simulink model "DCP_DCN_PWM"  (R2013a)
settings: Solver=FixedStepDiscrete  SolverMode=SingleTasking  StartTime=0.0  StopTime=inf  FixedStep=Tpas  RelTol=1e-3
undefined symbols (not defined in the file): fmod4Q, IDCP, KLPDCP, L, Lcoup, PDCP, R, TLPDCP, Tpas, Vdc
libraries: powerlib x51, simulink x15, powerlib_meascontrol x4
settings Model: Creator=LiberT  LastModifiedBy=Francis
settings DataIOCC: SignalLoggingSaveFormat=ModelDataLogs
settings OptimizationCC: ExpressionDepthLimit=2147483647
settings DebuggingCC: MultiTaskDSMMsg=warning  MultiTaskCondExecSysMsg=none  FcnCallInpInsideContextMsg=EnableAllAsWarning  StrictBusMsg=None
settings RTWCC: IncludeERTFirstTime=on

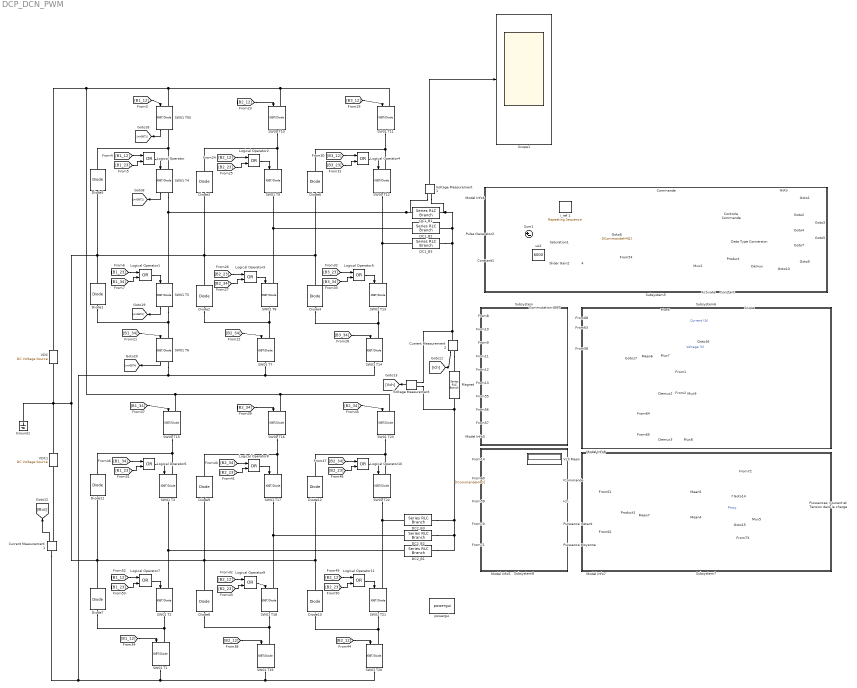
== system DCP_DCN_PWM ==
  " " : ManualSwitch
  " 4" : ManualSwitch  CurrentSetting=0
  Activate : Constant  Value=0
  Commande : Subsystem
  Commutation IGBT : Scope  NumInputPorts=9
      settings: TickLabels=on  TimeRange=0.04  YMin=-0.2~-0.2~-0.2~-0.2~-0.2~-0.2~-0.2~-0.2~-0.2  YMax=1.2~1.2~1.2~1.2~1.2~1.2~1.2~1.2~1.2
  Constant : Constant  Value=[1 1 1 1 1 1 1 1 1]
  Constant1 : Constant  Value=6000
  Controle Commande : ManualSwitch
  Current Measurement1 : powerlib/Measurements/Current Measurement  PhasorSimulation=off  OutputType=Complex  PSBequivalent=0
  Current Measurement2 : powerlib/Measurements/Current Measurement  PhasorSimulation=off  OutputType=Complex  PSBequivalent=0
  DC1_B1 : powerlib/Elements/Series RLC Branch  LConnTagsString=__new0  RConnTagsString=__new0  BranchType=L  Resistance=0  Inductance=Lcoup  SetiL0=off  InitialCurrent=0  Capacitance=1e-6  Setx0=off  InitialVoltage=0  Measurements=Branch current
  DC1_B2 : powerlib/Elements/Series RLC Branch  LConnTagsString=__new0  RConnTagsString=__new0  BranchType=L  Resistance=0  Inductance=Lcoup  SetiL0=off  InitialCurrent=0  Capacitance=1e-6  Setx0=off  InitialVoltage=0  Measurements=Branch current
  DC1_B3 : powerlib/Elements/Series RLC Branch  LConnTagsString=__new0  RConnTagsString=__new0  BranchType=L  Resistance=0  Inductance=Lcoup  SetiL0=off  InitialCurrent=0  Capacitance=1e-6  Setx0=off  InitialVoltage=0  Measurements=Branch current
  "DC2_B1 " : powerlib/Elements/Series RLC Branch  LConnTagsString=__new0  RConnTagsString=__new0  BranchType=L  Resistance=0  Inductance=Lcoup  SetiL0=off  InitialCurrent=0  Capacitance=1e-6  Setx0=off  InitialVoltage=0  Measurements=Branch current
  DC2_B2 : powerlib/Elements/Series RLC Branch  LConnTagsString=__new0  RConnTagsString=__new0  BranchType=L  Resistance=0  Inductance=Lcoup  SetiL0=off  InitialCurrent=0  Capacitance=1e-6  Setx0=off  InitialVoltage=0  Measurements=Branch current
  DC2_B3 : powerlib/Elements/Series RLC Branch  LConnTagsString=__new0  RConnTagsString=__new0  BranchType=L  Resistance=0  Inductance=Lcoup  SetiL0=off  InitialCurrent=0  Capacitance=1e-6  Setx0=off  InitialVoltage=0  Measurements=Branch current
  Data Type Conversion : DataTypeConversion  OutDataTypeStr=boolean
  Demux : Demux  Outputs=9
  Demux2 : Demux  Outputs=2
  Demux3 : Demux  Outputs=2
  Diode{1..12} (12 alike) : powerlib/Power Electronics/Diode  Ron=0.001  Lon=0  Vf=0.8  IC=0  UseSnubber=off  Rs=500  Cs=inf  Measurements=off
  Ground1 : powerlib/Elements/Ground  LConnTagsString=a
  ICommande : Display
  Ich : Display
  Logical Operator{,1..11} (12 alike) : Logic  Operator=OR  AllPortsSameDT=off  OutDataTypeStr=boolean
  Magnet : powerlib/Elements/Series RLC Branch  LConnTagsString=__new0  RConnTagsString=__new0  BranchType=RL  Resistance=R  Inductance=L  SetiL0=off  InitialCurrent=0  Capacitance=1e-6  Setx0=off  InitialVoltage=0  Measurements=Branch voltage and current
  Mean4 : powerlib_meascontrol/Measurements/Mean  Freq=1/.9  Vinit=0  Ts=Tpas
  Mean5 : powerlib_meascontrol/Measurements/Mean  Freq=fmod4Q  Vinit=0  Ts=Tpas
  Mean6 : powerlib_meascontrol/Measurements/Mean  Freq=fmod4Q/3  Vinit=0  Ts=Tpas
  Mean7 : powerlib_meascontrol/Measurements/Mean  Freq=fmod4Q/2  Vinit=0  Ts=Tpas
  Model Info{3,5,7..8} (4 alike) : simulink/Model-Wide Utilities/Model Info  InitialBlockCM=None  BlockCM=None  Frame=on  DisplayStringWithTags=Résultats  HorizontalTextAlignment=Center  LeftAlignmentValue=0.5  SourceBlockDiagram=DCP_DCN_PWM  TagMaxNumber=20
  Model Info6 : simulink/Model-Wide Utilities/Model Info  InitialBlockCM=None  BlockCM=None  Frame=on  DisplayStringWithTags=Commande H4Q  HorizontalTextAlignment=Center  LeftAlignmentValue=0.5  SourceBlockDiagram=DCP_DCN_PWM  TagMaxNumber=20
  Mux2 : Mux  Inputs=9
  Mux{5..9} (5 alike) : Mux  Inputs=2
  Product : Product
  Product1 : Product
  Puissance Instant. : Display
  Puissance Moyenne : Display
  "Puissances, Courant et Tension dans la charge" : Scope  NumInputPorts=3
      settings: TickLabels=on  TimeRange=0.9  YMin=-100~-25000000~-5000  YMax=6200~25000000~4500  SaveName=ScopeData4
  Pulse Generator2 : DiscretePulseGenerator  Amplitude=12000  Period=floor(.4 /Tpas)  PulseWidth=floor(.4 * .5 / Tpas)  PhaseDelay=floor(.001 / Tpas)  SampleTime=Tpas
  SW01 T05 : powerlib/Power Electronics/IGBT//Diode  Ron=Ron  Rs=Rs  Cs=Cs  Measurements=on
  SW01 T{1..3,7..23} (20 alike) : powerlib/Power Electronics/IGBT//Diode  Ron=Ron  Rs=Rs  Cs=Cs  Measurements=off
  SW01 T4 : powerlib/Power Electronics/IGBT//Diode  Ron=Ron  Rs=Rs  Cs=Cs  Measurements=on
  SW01 T5 : powerlib/Power Electronics/IGBT//Diode  Ron=Ron  Rs=Rs  Cs=Cs  Measurements=on
  SW01 T6 : powerlib/Power Electronics/IGBT//Diode  Ron=Ron  Rs=Rs  Cs=Cs  Measurements=on
  Saturation1 : Saturate  UpperLimit=5000  LowerLimit=2000
  Scope : Scope  NumInputPorts=6
      settings: TimeRange=0.9  YMin=-7000~-5000~-0.1~-0.1~-15000~0  YMax=7000~5000~1.1~1.1~15000~2500  SaveName=ScopeData5  MaxDataPoints=10000
  Scope1 : Scope
      settings: TimeRange=0.9  YMin=-7000  YMax=7000  SaveName=ScopeData6  MaxDataPoints=10000
  Slider Gain2 : simulink/Math Operations/Slider Gain  low=0  gain=0.54  high=1
  Subsystem : Subsystem
      mask Display: disp('')
  Subsystem5 : Subsystem
      mask Display: disp('')
  Subsystem6 : Subsystem
      mask Display: disp('')
  Subsystem7 : Subsystem
      mask Display: disp('')
  Subsystem8 : Subsystem
      mask Display: disp('')
  Sum1 : Sum  Inputs=|+-
  VDC : powerlib/Electrical Sources/DC Voltage Source  Amplitude=Vdc/2  Measurements=None
  VDC1 : powerlib/Electrical Sources/DC Voltage Source  Amplitude=Vdc/2  Measurements=None
  Vch Mean : Display
  Voltage Measurement : powerlib/Measurements/Voltage Measurement  PhasorSimulation=off  OutputType=Complex  PSBequivalent=0
  Voltage Measurement1 : powerlib/Measurements/Voltage Measurement  PhasorSimulation=off  OutputType=Complex  PSBequivalent=0
  i_ref 1 : simulink/Sources/Repeating Sequence  rep_seq_t="[0 108.51e-3 127.6e-3 132e-3 200e-3 250e-3 283.33e-3 310e-3 366.66e-3  490e-3 533e-3 683.33e-3 900e-3]"  rep_seq_y=[333 333 1000 1031 1500 2000 2500 3000 4000 6000 6000 333 333]
  powergui : powerlib/powergui  Priority=1  SimulationMode=Discrete  SolverType=Tustin  SampleTime=Tpas  frequency=60  SPID=off  DisableSnubberDevices=off  DisableRonSwitches=off  DisableVfSwitches=off  SwTol=0  Interpol=off  DisplayEquations=off  frequencyindice=0  Pbase=100e6  ErrMax=1e-4  Iterations=50  UnitsV=kV  UnitsW=MW  FunctionMessages=off  echomessages=off  HookPort=off  EnableUseOfTLC=off  x0status=blocks  RestoreLinks=warning  ResistiveCurrentMeasurement=off  Frange=[0:2:500]  Ylog=off  Xlog=on  ShowGrid=off  save=off  variable=ZData  structure=ScopeData6  ZoomFFT=off  StartTime=3.7  cycles=130  DisplayStyle=1  fundamental=333  FreqAxis=on  MaxFrequency=2000  frequencyindicesteady=1  RmsSteady=1  display=off  Ts=0  methode=off
  uo2 : Constant  Value=6000
  wires:
  [B1_12] -> Commutation IGBT/1
  [B1_23] -> Commutation IGBT/2
  [B1_34] -> Commutation IGBT/3
  [B2_12] -> Commutation IGBT/4
  [B2_23] -> Commutation IGBT/5
  [B2_34] -> Commutation IGBT/6
  Constant/1 -> Product/2
  Activate/1 -> Product/1
  Controle Commande/1 -> Demux/1
  Mux2/1 -> Controle Commande/1
  Data Type Conversion/1 -> Controle Commande/2
  Product/1 -> Data Type Conversion/1
  Commande/1(12_B1) -> Mux2/1
  Commande/2(23_B1) -> Mux2/2
  Commande/3(34_B1) -> Mux2/3
  Demux/1 -> [B1_12]
  Demux/3 -> [B1_34]
  Demux/2 -> [B1_23]
  [B1_12] -> SW01 T05/1
  Logical Operator/1 -> SW01 T4/1
  [B1_12] -> Logical Operator/1
  [B1_23] -> Logical Operator/2
  Logical Operator1/1 -> SW01 T5/1
  [B1_23] -> Logical Operator1/1
  [B1_34] -> Logical Operator1/2
  [B1_34] -> SW01 T6/1
  [B2_12] -> SW01 T10/1
  Logical Operator2/1 -> SW01 T9/1
  [B2_12] -> Logical Operator2/1
  [B2_23] -> Logical Operator2/2
  Logical Operator3/1 -> SW01 T8/1
  [B2_23] -> Logical Operator3/1
  [B2_34] -> Logical Operator3/2
  [B2_34] -> SW01 T7/1
  [B3_12] -> SW01 T11/1
  Logical Operator4/1 -> SW01 T12/1
  [B3_12] -> Logical Operator4/1
  [B3_23] -> Logical Operator4/2
  Logical Operator5/1 -> SW01 T13/1
  [B3_23] -> Logical Operator5/1
  [B3_34] -> Logical Operator5/2
  [B3_34] -> SW01 T14/1
  [B1_34] -> SW01 T15/1
  Logical Operator6/1 -> SW01 T3/1
  [B1_34] -> Logical Operator6/1
  [B1_23] -> Logical Operator6/2
  Logical Operator7/1 -> SW01 T2/1
  [B1_12] -> Logical Operator7/1
  [B1_23] -> Logical Operator7/2
  [B1_12] -> SW01 T1/1
  [B2_34] -> SW01 T16/1
  Logical Operator8/1 -> SW01 T17/1
  [B2_34] -> Logical Operator8/1
  [B2_23] -> Logical Operator8/2
  Logical Operator9/1 -> SW01 T18/1
  [B2_12] -> Logical Operator9/1
  [B2_23] -> Logical Operator9/2
  [B2_12] -> SW01 T19/1
  [B2_34] -> SW01 T23/1
  Logical Operator10/1 -> SW01 T22/1
  [B2_34] -> Logical Operator10/1
  [B2_23] -> Logical Operator10/2
  Logical Operator11/1 -> SW01 T21/1
  [B2_12] -> Logical Operator11/1
  [B2_23] -> Logical Operator11/2
  [B2_12] -> SW01 T20/1
  Current Measurement1/1 -> [IBus]
  uo2/1 -> Slider Gain2/1
  Slider Gain2/1 -> " 4"/2
  Saturation1/1 -> " 4"/1
  Constant1/1 -> Sum1/2
  i_ref 1/1 -> " "/1
  " 4"/1 -> " "/2
  Pulse Generator2/1 -> Sum1/1
  Sum1/1 -> Saturation1/1
  " "/1 -> Commande/1(Iref), [ICommandeH4Q]
  Commande/4(12_B2) -> Mux2/4
  Commande/5(23_B2) -> Mux2/5
  Commande/6(34_B2) -> Mux2/6
  Commande/7(12_B3) -> Mux2/7
  Commande/8(23_B3) -> Mux2/8
  Commande/9(34_B3) -> Mux2/9
  Demux/4 -> [B2_12]
  Demux/6 -> [B2_34]
  Demux/5 -> [B2_23]
  Demux/7 -> [B3_12]
  Demux/9 -> [B3_34]
  Demux/8 -> [B3_23]
  Current Measurement2/1 -> [Ich]
  Voltage Measurement/1 -> [Vch]
  [Ich] -> Commande/2("Iload ")
  [B3_12] -> Commutation IGBT/7
  [B3_23] -> Commutation IGBT/8
  [B3_34] -> Commutation IGBT/9
  [Ich] -> Ich/1
  [VMeanLoad] -> Vch Mean/1
  [ICommandeH4Q] -> ICommande/1
  [P] -> Puissance Instant./1
  [Pmoy] -> Puissance Moyenne/1
  Mean4/1 -> [Pmoy], Mux5/2  "Pmoy"
  Mean5/1 -> [P], Mux5/1  "P"
  Mux6/1 -> [IScope], Scope/1  "Current (A)"
  Mux7/1 -> Scope/2  "Voltage (V)"
  [Ich] -> Mux6/2
  [mIGBT1] -> Demux2/1
  Mean6/1 -> [VMeanLoad], Mux7/2
  [Vch] -> Mux7/1, Mean6/1
  [mIGBT2] -> Demux3/1
  [B1_12] -> Scope/3
  Mux8/1 -> Scope/6
  Mux9/1 -> Scope/5
  [B1_34] -> Scope/4
  Demux2/1 -> Mux9/1
  Demux3/1 -> Mux9/2
  Demux2/2 -> Mux8/1
  Demux3/2 -> Mux8/2
  [ICommandeH4Q] -> Mux6/1
  [Vch] -> Product1/1
  [Ich] -> Product1/2
  Product1/1 -> Mean7/1
  Mean7/1 -> Mean4/1, Mean5/1
  Mux5/1 -> "Puissances, Courant et Tension dans la charge"/2
  [IScope] -> "Puissances, Courant et Tension dans la charge"/1
  [VMeanLoad] -> "Puissances, Courant et Tension dans la charge"/3
  SW01 T4/1 -> [mIGBT2]
  SW01 T05/1 -> [mIGBT1]
  SW01 T5/1 -> [mIGBT3]
  SW01 T6/1 -> [mIGBT4]
  Voltage Measurement1/1 -> Scope1/1
  connections:
  DC1_B1/LConn1 -- SW01 T5/LConn1 -- SW01 T4/RConn1 -- Voltage Measurement1/LConn1
  DC1_B3/LConn1 -- SW01 T13/LConn1 -- SW01 T12/RConn1
  DC1_B2/LConn1 -- SW01 T9/RConn1 -- SW01 T8/LConn1
  Diode5/RConn1 -- SW01 T05/RConn1 -- SW01 T4/LConn1
  Diode3/RConn1 -- SW01 T10/RConn1 -- SW01 T9/LConn1
  Diode6/RConn1 -- SW01 T12/LConn1 -- SW01 T11/RConn1
  Diode1/LConn1 -- SW01 T6/LConn1 -- SW01 T5/RConn1
  Diode4/LConn1 -- SW01 T14/LConn1 -- SW01 T13/RConn1
  Diode2/LConn1 -- SW01 T8/RConn1 -- SW01 T7/LConn1
  SW01 T1/RConn1 -- Current Measurement1/LConn1 -- SW01 T6/RConn1 -- SW01 T14/RConn1 -- SW01 T7/RConn1 -- SW01 T20/RConn1 -- SW01 T19/RConn1
  SW01 T15/LConn1 -- SW01 T11/LConn1 -- SW01 T10/LConn1 -- SW01 T05/LConn1 -- VDC/RConn1 -- SW01 T23/LConn1 -- SW01 T16/LConn1
  Diode11/RConn1 -- SW01 T15/RConn1 -- SW01 T3/LConn1
  Diode9/RConn1 -- SW01 T17/LConn1 -- SW01 T16/RConn1
  Diode12/RConn1 -- SW01 T23/RConn1 -- SW01 T22/LConn1
  Diode7/LConn1 -- SW01 T2/RConn1 -- SW01 T1/LConn1
  Diode10/LConn1 -- SW01 T21/RConn1 -- SW01 T20/LConn1
  Diode8/LConn1 -- SW01 T19/LConn1 -- SW01 T18/RConn1
  Ground1/LConn1 -- Diode4/RConn1 -- Diode6/LConn1 -- Diode3/LConn1 -- Diode2/RConn1 -- Diode5/LConn1 -- Diode1/RConn1 -- Diode11/LConn1 -- Diode7/RConn1 -- Diode9/LConn1 -- Diode8/RConn1 -- Diode10/RConn1 -- Diode12/LConn1 -- VDC/LConn1 -- VDC1/RConn1
  SW01 T21/LConn1 -- DC2_B3/RConn1 -- SW01 T22/RConn1
  SW01 T2/LConn1 -- "DC2_B1 "/RConn1 -- SW01 T3/RConn1
  SW01 T17/RConn1 -- DC2_B2/RConn1 -- SW01 T18/LConn1
  Current Measurement1/RConn1 -- VDC1/LConn1
  DC1_B1/RConn1 -- Voltage Measurement/LConn1 -- Current Measurement2/LConn1 -- DC1_B3/RConn1 -- DC1_B2/RConn1 -- Voltage Measurement1/LConn2
  DC2_B3/LConn1 -- "DC2_B1 "/LConn1 -- DC2_B2/LConn1 -- Voltage Measurement/LConn2 -- Magnet/RConn1
  Current Measurement2/RConn1 -- Magnet/LConn1

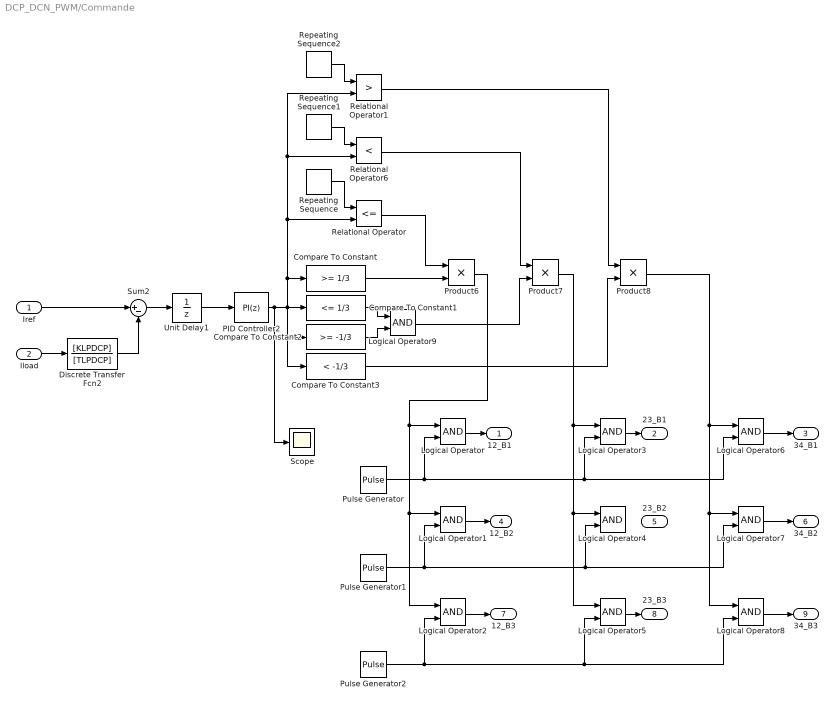
== system DCP_DCN_PWM/Commande ==
  Iref : Inport
  "Iload " : Inport  Port=2
  Compare To Constant : simulink/Logic and Bit Operations/Compare To Constant  relop=>=  const=1/3  OutDataTypeStr=boolean
  Compare To Constant1 : simulink/Logic and Bit Operations/Compare To Constant  relop=<=  const=1/3  OutDataTypeStr=boolean
  Compare To Constant2 : simulink/Logic and Bit Operations/Compare To Constant  relop=>=  const=-1/3  OutDataTypeStr=boolean
  Compare To Constant3 : simulink/Logic and Bit Operations/Compare To Constant  relop=<  const=-1/3  OutDataTypeStr=boolean
  Discrete Transfer Fcn2 : DiscreteTransferFcn  Numerator=[KLPDCP]  Denominator=[TLPDCP]  SampleTime=Tpas
  Logical Operator{,1..9} (10 alike) : Logic  AllPortsSameDT=off  OutDataTypeStr=boolean  SampleTime=Tpas
  PID Controller2 : simulink/Continuous/PID Controller  Controller=PI  TimeDomain=Discrete-time  SampleTime=Tpas  IntegratorMethod=Forward Euler  FilterMethod=Forward Euler  Form=Parallel  P=PDCP  I=IDCP  D=0  N=100  InitialConditionSource=internal  InitialConditionForIntegrator=0  InitialConditionForFilter=0  ExternalReset=none  LimitOutput=on  UpperSaturationLimit=1  LowerSaturationLimit=-1  LinearizeAsGain=on  AntiWindupMode=clamping  Kb=1  TrackingMode=off  Kt=1  PParamMin=[]  PParamMax=[]  IParamMin=[]  IParamMax=[]  DParamMin=[]  DParamMax=[]  NParamMin=[]  NParamMax=[]  KbParamMin=[]  KbParamMax=[]  KtParamMin=[]  KtParamMax=[]  POutMin=[]  POutMax=[]  IOutMin=[]  IOutMax=[]  DOutMin=[]  DOutMax=[]  NOutMin=[]  NOutMax=[]  KbOutMin=[]  KbOutMax=[]  KtOutMin=[]  KtOutMax=[]  IntegratorOutMin=[]  IntegratorOutMax=[]  FilterOutMin=[]  FilterOutMax=[]  SumOutMin=[]  SumOutMax=[]  SumI1OutMin=[]  SumI1OutMax=[]  SumI2OutMin=[]  SumI2OutMax=[]  SumI3OutMin=[]  SumI3OutMax=[]  SumDOutMin=[]  SumDOutMax=[]  SaturationOutMin=[]  SaturationOutMax=[]  IntegratorContinuousStateAttributes=''  IntegratorStateMustResolveToSignalObject=off  IntegratorRTWStateStorageClass=Auto  FilterContinuousStateAttributes=''  FilterStateMustResolveToSignalObject=off  FilterRTWStateStorageClass=Auto
  Product6 : Product  SampleTime=Tpas
  Product7 : Product  SampleTime=Tpas
  Product8 : Product  SampleTime=Tpas
  Pulse Generator : DiscretePulseGenerator  Period=floor(1/(fmod4Q/3) * 1/Tpas)  PulseWidth=floor(1/(fmod4Q) * 1/Tpas)  SampleTime=Tpas
  Pulse Generator1 : DiscretePulseGenerator  Period=floor(1/(fmod4Q/3) * 1/Tpas)  PulseWidth=floor(1/(fmod4Q) * 1/Tpas)  PhaseDelay=floor(1/(fmod4Q) * 1/Tpas)  SampleTime=Tpas
  Pulse Generator2 : DiscretePulseGenerator  Period=floor(1/(fmod4Q/3) * 1/Tpas)  PulseWidth=floor(1/(fmod4Q) * 1/Tpas)  PhaseDelay=floor(2/(fmod4Q) * 1/Tpas)  SampleTime=Tpas
  Relational Operator : RelationalOperator  Operator=<=  OutDataTypeStr=boolean
  Relational Operator1 : RelationalOperator  Operator=>  OutDataTypeStr=boolean
  Relational Operator6 : RelationalOperator  Operator=<  OutDataTypeStr=boolean
  Repeating Sequence : simulink/Sources/Repeating Sequence  rep_seq_t=[0 1/fmod4Q]  rep_seq_y=[1/3 1.035]
  Repeating Sequence1 : simulink/Sources/Repeating Sequence  rep_seq_t=[0 1/fmod4Q]  rep_seq_y=[-.35 .35]
  Repeating Sequence2 : simulink/Sources/Repeating Sequence  rep_seq_t=[0 1/fmod4Q]  rep_seq_y=[-1 -1/3]
  Scope : Scope
      settings: SaveName=ScopeData3
  Sum2 : Sum  Inputs=|+-
  Unit Delay1 : UnitDelay  SampleTime=-1
  12_B1 : Outport
  23_B1 : Outport  Port=2
  34_B1 : Outport  Port=3
  12_B2 : Outport  Port=4
  23_B2 : Outport  Port=5
  34_B2 : Outport  Port=6
  12_B3 : Outport  Port=7
  23_B3 : Outport  Port=8
  34_B3 : Outport  Port=9
  wires:
  Compare To Constant/1 -> Product6/2
  Compare To Constant3/1 -> Product8/2
  Compare To Constant1/1 -> Logical Operator9/1
  Compare To Constant2/1 -> Logical Operator9/2
  Logical Operator9/1 -> Product7/2
  Repeating Sequence/1 -> Relational Operator/1
  Repeating Sequence2/1 -> Relational Operator1/1
  Relational Operator/1 -> Product6/1
  Relational Operator6/1 -> Product7/1
  Relational Operator1/1 -> Product8/1
  PID Controller2/1 -> Scope/1, Relational Operator/2, Relational Operator1/2, Relational Operator6/2, Compare To Constant/1, Compare To Constant1/1, Compare To Constant3/1, Compare To Constant2/1
  Repeating Sequence1/1 -> Relational Operator6/1
  Iref/1 -> Sum2/1
  "Iload "/1 -> Discrete Transfer Fcn2/1
  Discrete Transfer Fcn2/1 -> Sum2/2
  Sum2/1 -> Unit Delay1/1
  Unit Delay1/1 -> PID Controller2/1
  Product6/1 -> Logical Operator2/1, Logical Operator1/1, Logical Operator/1
  Pulse Generator2/1 -> Logical Operator5/2, Logical Operator8/2, Logical Operator2/2
  Pulse Generator/1 -> Logical Operator3/2, Logical Operator6/2, Logical Operator/2
  Pulse Generator1/1 -> Logical Operator1/2, Logical Operator4/2, Logical Operator7/2
  Product7/1 -> Logical Operator5/1, Logical Operator4/1, Logical Operator3/1
  Product8/1 -> Logical Operator8/1, Logical Operator7/1, Logical Operator6/1
  Logical Operator/1 -> 12_B1/1
  Logical Operator8/1 -> 34_B3/1
  Logical Operator1/1 -> 12_B2/1
  Logical Operator3/1 -> 23_B1/1
  Logical Operator6/1 -> 34_B1/1
  Logical Operator2/1 -> 12_B3/1
  Logical Operator5/1 -> 23_B3/1
  Logical Operator7/1 -> 34_B2/1

== system DCP_DCN_PWM/Subsystem ==

== system DCP_DCN_PWM/Subsystem5 ==

== system DCP_DCN_PWM/Subsystem6 ==

== system DCP_DCN_PWM/Subsystem7 ==

== system DCP_DCN_PWM/Subsystem8 ==
